simulink model "OMC_for_RDTS"  (R2019b)
settings: Solver=ode8  StartTime=0.0  StopTime=50  FixedStep=1  RelTol=1e-3
values from neighbouring files (symbols this model uses):
  A = sssys_d.A    [RTDS2022.m]
  B = sssys_d.B    [RTDS2022.m]
  C = sssys_d.C    [RTDS2022.m]
  K = place(A, B, z_desired_system)    [RTDS2022.m]
  L = L_tr'    [RTDS2022.m]
  T = 1    [RTDS2022.m]
  v0 = [0; 0]    [RTDS2022.m]
  x0 = [5; -5]    [RTDS2022.m]
settings Model: Creator=Aleksandr Gogotov  LastModifiedBy=Aleksandr Gogotov
settings DataIOCC: ReturnWorkspaceOutputs=off
settings DebuggingCC: ArithmeticOperatorsInVariantConditions=warning
settings SFSimCC: SimUseLocalCustomCode=off  CustomCodeUndefinedFunction=UseInterfaceOnly
settings RTWCC: RTWUseLocalCustomCode=off

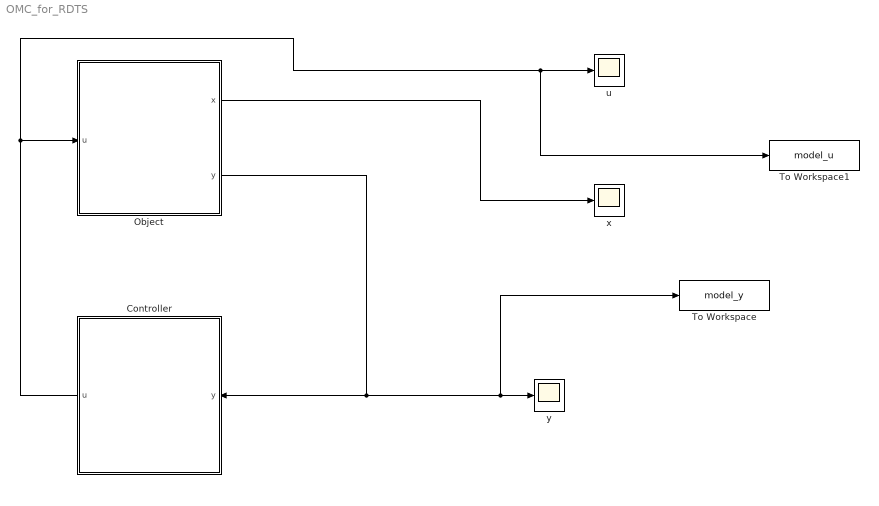
== system OMC_for_RDTS ==
  Controller : Subsystem
  "Object " : Subsystem
  To Workspace : ToWorkspace  VariableName=model_y  SampleTime=T
      settings: Save2DSignal=2-D array (concatenate along first dimension)
  To Workspace1 : ToWorkspace  VariableName=model_u  SampleTime=T
      settings: Save2DSignal=2-D array (concatenate along first dimension)
  "u " : Scope
  x : Scope
  y : Scope
  wires:
  Controller/1("u ") -> To Workspace1/1, "u "/1, "Object "/1("u ")
  "Object "/2("y ") -> To Workspace/1, y/1, Controller/1("y ")
  "Object "/1("x ") -> x/1

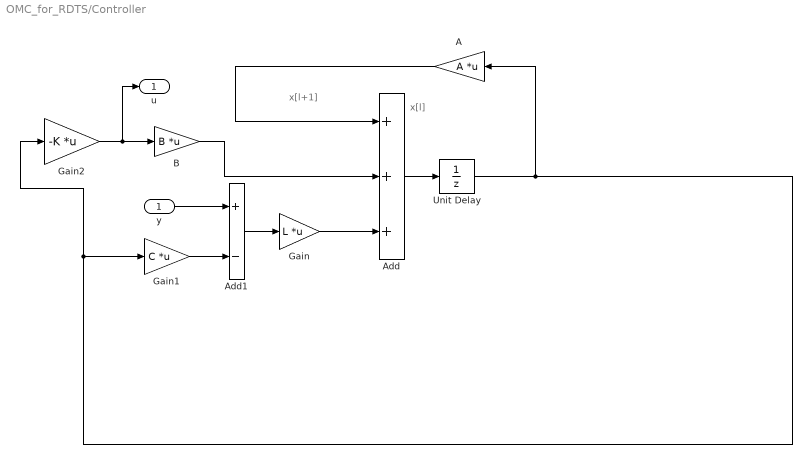
== system OMC_for_RDTS/Controller ==
  note: x[l]
  note: x[l+1]
  "y " : Inport
  "A " : Gain  Gain=A  Multiplication=Matrix(K*u)
  Add : Sum  Inputs=+++
  Add1 : Sum  Inputs=+-
  B : Gain  Gain=B  Multiplication=Matrix(K*u)
  Gain : Gain  Gain=L  Multiplication=Matrix(K*u)
  Gain1 : Gain  Gain=C  Multiplication=Matrix(K*u)
  Gain2 : Gain  Gain=-K  Multiplication=Matrix(K*u)
  Unit Delay : UnitDelay  InitialCondition=v0  SampleTime=T  HasFrameUpgradeWarning=on
  "u " : Outport
  wires:
  "A "/1 -> Add/1
  B/1 -> Add/2
  Add/1 -> Unit Delay/1
  Gain2/1 -> "u "/1, B/1
  Unit Delay/1 -> "A "/1, Gain2/1, Gain1/1
  Gain/1 -> Add/3
  Add1/1 -> Gain/1
  "y "/1 -> Add1/1
  Gain1/1 -> Add1/2

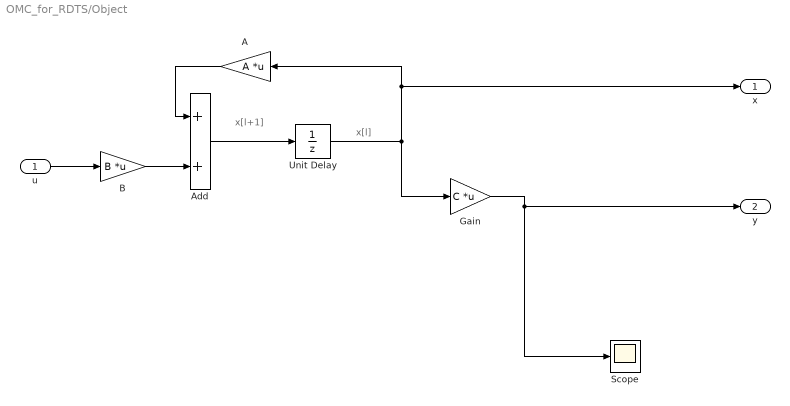
== system OMC_for_RDTS/Object  ==
  note: x[l]
  note: x[l+1]
  "u " : Inport
  "A " : Gain  Gain=A  Multiplication=Matrix(K*u)
  Add : Sum
  B : Gain  Gain=B  Multiplication=Matrix(K*u)
  Gain : Gain  Gain=C  Multiplication=Matrix(K*u)
  Scope : Scope
  Unit Delay : UnitDelay  InitialCondition=x0  SampleTime=T  HasFrameUpgradeWarning=on
  "x " : Outport  VectorParamsAs1DForOutWhenUnconnected=off
  "y " : Outport  Port=2  VectorParamsAs1DForOutWhenUnconnected=off
  wires:
  "A "/1 -> Add/1
  B/1 -> Add/2
  Add/1 -> Unit Delay/1
  "u "/1 -> B/1
  Gain/1 -> "y "/1, Scope/1
  Unit Delay/1 -> Gain/1, "x "/1, "A "/1
